simulink model "drone_level_4"  (R2023a)
settings: Solver=VariableStepAuto  StartTime=0.0  StopTime=10.0  RelTol=1e-3
values from neighbouring files (symbols this model uses):
  Kp_omega = 10    [tuning.m]
  Kp_theta = 5.6    [tuning.m]
  Kp_vx = -0.2    [tuning.m]
  Kp_vy = 7.5    [tuning.m]
undefined symbols (not defined in the file or in its folder): dxdt
libraries: simulink x1
settings Model: Creator=timme  LastModifiedBy=timme
settings OptimizationCC: BlockReduction=off  DefaultParameterBehavior=Inlined  BufferReuse=off

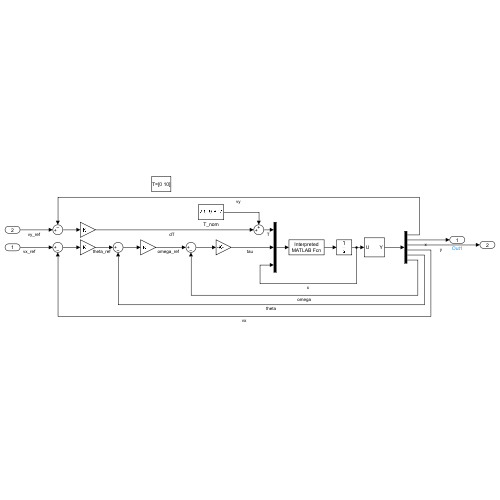
[thumbnail: Simulink's stored preview of the top-level diagram]
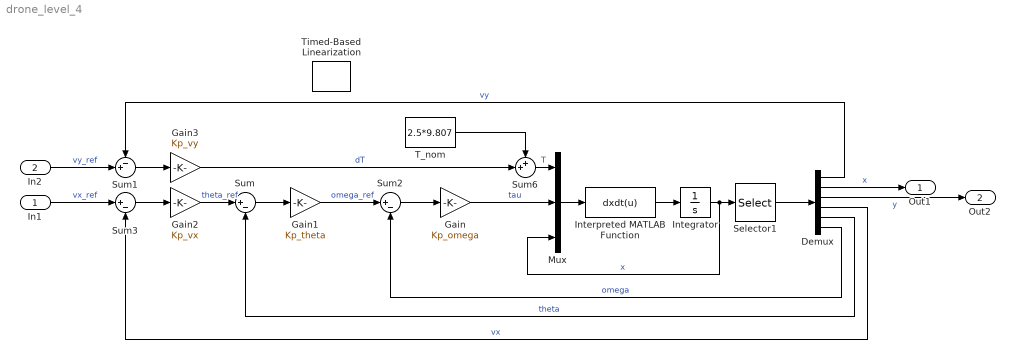
== system drone_level_4 ==
  In1 : Inport
  In2 : Inport  Port=2
  Demux : Demux  Outputs=6
  Gain : Gain  Gain=Kp_omega
  Gain1 : Gain  Gain=Kp_theta
  Gain2 : Gain  Gain=Kp_vx
  Gain3 : Gain  Gain=Kp_vy
  Integrator : Integrator  InitialCondition=zeros(6,1)
  Interpreted MATLAB Function : MATLABFcn  MATLABFcn=dxdt(u)  OutputDimensions=6
  Mux : Mux  Inputs=3
  Selector1 : Selector  InputPortWidth=6  IndexOptions=Index vector (dialog)  Indices=[5, 1, 2, 4, 3, 6]  OutputSizes=1
  Sum : Sum  Inputs=|+-
  Sum1 : Sum  Inputs=-+|
  Sum2 : Sum  Inputs=|+-
  Sum3 : Sum  Inputs=|+-
  Sum6 : Sum  Inputs=++|
  T_nom : Constant  Value=2.5*9.807
  Timed-Based Linearization : simulink/Model-Wide Utilities/Timed-Based Linearization  LinearizationTime=[0 10]  SampleTime=0
  Out1 : Outport
  Out2 : Outport  Port=2
  wires:
  Sum2/1 -> Gain/1
  Sum1/1 -> Gain3/1
  Selector1/1 -> Demux/1
  Mux/1 -> Interpreted MATLAB Function/1
  Interpreted MATLAB Function/1 -> Integrator/1
  Sum6/1 -> Mux/1  "T"
  Integrator/1 -> Selector1/1, Mux/3  "x"
  T_nom/1 -> Sum6/1
  Sum/1 -> Gain1/1
  Demux/6 -> Sum2/2  "omega"
  Demux/5 -> Sum/2  "theta"
  In1/1 -> Sum3/1  "vx_ref"
  Gain/1 -> Mux/2  "tau"
  Gain1/1 -> Sum2/1  "omega_ref"
  Demux/1 -> Sum1/1  "vy"
  In2/1 -> Sum1/2  "vy_ref"
  Demux/4 -> Sum3/2  "vx"
  Gain2/1 -> Sum/1  "theta_ref"
  Gain3/1 -> Sum6/2  "dT"
  Sum3/1 -> Gain2/1
  Demux/2 -> Out1/1  "x"
  Demux/3 -> Out2/1  "y"
